simulink model "Model_after"  (R2013b)
settings: Solver=ode45  StartTime=0.0  StopTime=10.0  RelTol=1e-3
settings Model: Creator=qiji  LastModifiedBy=qiji

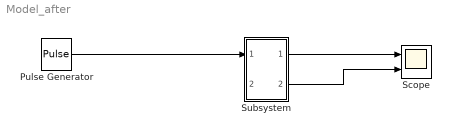
== system Model_after ==
  Pulse Generator : DiscretePulseGenerator  Period=5
  Scope : Scope  NumInputPorts=2
      settings: YMin=-5~-5  YMax=5~5
  Subsystem : Subsystem
  wires:
  Pulse Generator/1 -> Subsystem/1(In1)
  Subsystem/1(Out1) -> Scope/1
  Subsystem/2(Out2) -> Scope/2

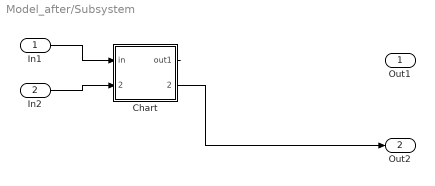
== system Model_after/Subsystem ==
  In1 : Inport
  In2 : Inport  Port=2
  Chart : Stateflow chart  TreatAsAtomicUnit=on
  Out1 : Outport
  Out2 : Outport  Port=2
  wires:
  Chart/2 -> Out2/1
  ?8/1 -> Out1/1
  Chart/1(out) -> ?8/1
  In1/1 -> Chart/1(in1)
  In2/1 -> Chart/2

== stateflow chart Model_after/Subsystem/Chart ==
  state Subsystem_Chart [parallel]
    settings: executionOrder=1
    state A
      en:
      out = 0;
      out1 = 0;
    state B
      en:
      out = 1;
      out1 =1;
    Subsystem_Chart.A -> B : [in == 1]
    (default) -> Subsystem_Chart.A
    B -> Subsystem_Chart.A : [in==1]
  state Subsystem_Chart1 [parallel]
    settings: executionOrder=1
    state A
      du:
      out = in
    (default) -> Subsystem_Chart1.A
  data: out output double; Subsystem/Chart/in input double; Subsystem/Chart/out1 output double; Subsystem/Chart/in1 input double; in input double; Subsystem/Chart1/out output double
